simulink model "Project3b"  (R2016a)
settings: Solver=ode5  StartTime=0.0  StopTime=tf  FixedStep=0.001  RelTol=1e-3
values from neighbouring files (symbols this model uses):
  k1 = 1    [Project3_FullCode.m]    (also in Project3a_Code.m = 30; Project3b_Code.m)
  k2 = 1    [Project3_FullCode.m]    (also in Project3a_Code.m = 40; Project3b_Code.m)
  ugain = 1    [Project3_FullCode.m]    (also in Project3a_Code.m; Project3b_Code.m)
  x10 = 0    [Project3_FullCode.m]    (also in Project3a_Code.m = 1; Project3b_Code.m)
  x20 = 2    [Project3_FullCode.m]    (also in Project3a_Code.m = 0; Project3b_Code.m)
settings Model: Creator=Dell  LastModifiedBy=Dell
settings DataIOCC: SaveFormat=Array

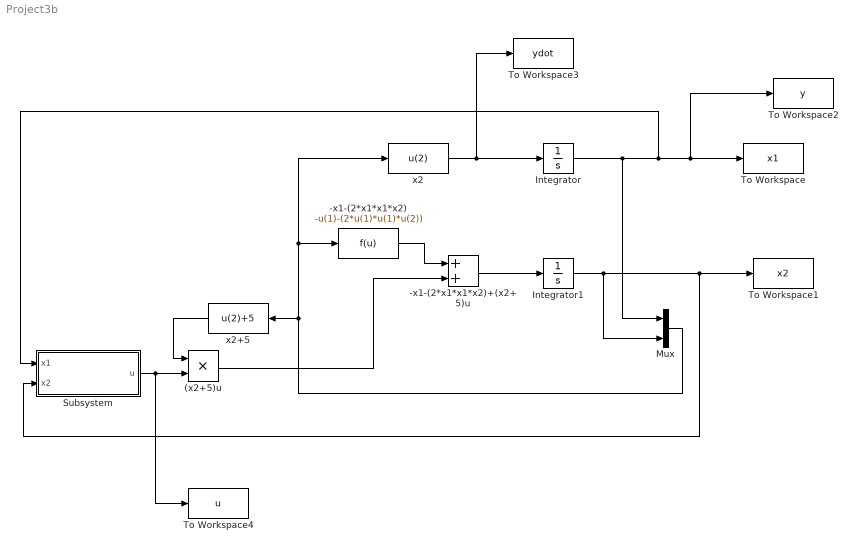
== system Project3b ==
  (x2+5)u : Product
  -x1-(2*x1*x1*x2) : Fcn  Expr=-u(1)-(2*u(1)*u(1)*u(2))
  -x1-(2*x1*x1*x2)+(x2+5)u : Sum
  Integrator : Integrator  InitialCondition=x10
  Integrator1 : Integrator  InitialCondition=x20
  Mux : Mux  Inputs=2
  Subsystem : Subsystem
  To Workspace : ToWorkspace  VariableName=x1  SampleTime=-1
  To Workspace1 : ToWorkspace  VariableName=x2  SampleTime=-1
  To Workspace2 : ToWorkspace  VariableName=y  SampleTime=-1
  To Workspace3 : ToWorkspace  VariableName=ydot  SampleTime=-1
  To Workspace4 : ToWorkspace  VariableName=u  SampleTime=-1
  x2 : Fcn  Expr=u(2)
  x2+5 : Fcn  Expr=u(2)+5
  wires:
  Integrator/1 -> Mux/1, Subsystem/1(x1), To Workspace2/1, To Workspace/1
  Integrator1/1 -> Mux/2, Subsystem/2("x2 "), To Workspace1/1
  Mux/1 -> x2+5/1, -x1-(2*x1*x1*x2)/1, x2/1
  x2/1 -> To Workspace3/1, Integrator/1
  Subsystem/1(u) -> To Workspace4/1, (x2+5)u/2
  x2+5/1 -> (x2+5)u/1
  -x1-(2*x1*x1*x2)/1 -> -x1-(2*x1*x1*x2)+(x2+5)u/1
  (x2+5)u/1 -> -x1-(2*x1*x1*x2)+(x2+5)u/2
  -x1-(2*x1*x1*x2)+(x2+5)u/1 -> Integrator1/1

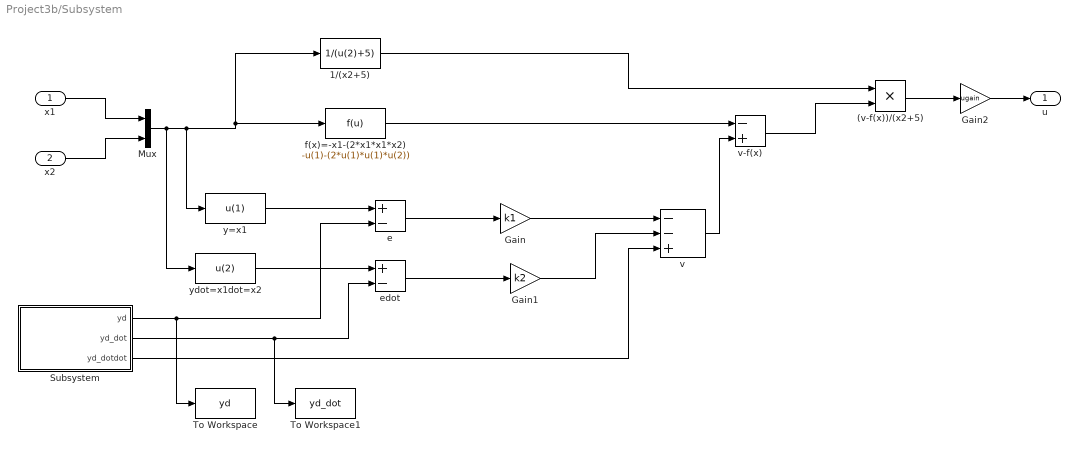
== system Project3b/Subsystem ==
  x1 : Inport
  "x2 " : Inport  Port=2
  (v-f(x))/(x2+5) : Product
  1/(x2+5) : Fcn  Expr=1/(u(2)+5)
  Gain : Gain  Gain=k1
  Gain1 : Gain  Gain=k2
  Gain2 : Gain  Gain=ugain
  Mux : Mux  Inputs=2
  Subsystem : Subsystem
  To Workspace : ToWorkspace  VariableName=yd  SampleTime=-1
  To Workspace1 : ToWorkspace  VariableName=yd_dot  SampleTime=-1
  e : Sum  Inputs=+-
  edot : Sum  Inputs=+-
  f(x)=-x1-(2*x1*x1*x2) : Fcn  Expr=-u(1)-(2*u(1)*u(1)*u(2))
  v : Sum  Inputs=--+
  v-f(x) : Sum  Inputs=-+
  y=x1 : Fcn  Expr=u(1)
  ydot=x1dot=x2 : Fcn  Expr=u(2)
  u : Outport
  wires:
  x1/1 -> Mux/1
  "x2 "/1 -> Mux/2
  Mux/1 -> ydot=x1dot=x2/1, y=x1/1, f(x)=-x1-(2*x1*x1*x2)/1, 1/(x2+5)/1
  y=x1/1 -> e/1
  Subsystem/1(yd) -> e/2, To Workspace/1
  ydot=x1dot=x2/1 -> edot/1
  Subsystem/2(yd_dot) -> To Workspace1/1, edot/2
  e/1 -> Gain/1
  edot/1 -> Gain1/1
  Gain/1 -> v/1
  Gain1/1 -> v/2
  Subsystem/3(yd_dotdot) -> v/3
  f(x)=-x1-(2*x1*x1*x2)/1 -> v-f(x)/1
  v/1 -> v-f(x)/2
  1/(x2+5)/1 -> (v-f(x))/(x2+5)/1
  v-f(x)/1 -> (v-f(x))/(x2+5)/2
  (v-f(x))/(x2+5)/1 -> Gain2/1
  Gain2/1 -> u/1

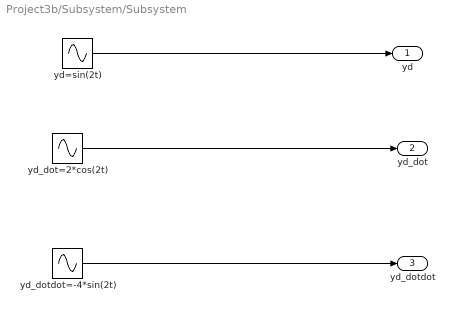
== system Project3b/Subsystem/Subsystem ==
  " yd=sin(2t)" : Sin  Frequency=2  SampleTime=0
  yd_dot=2*cos(2t) : Sin  Amplitude=2  Frequency=2  Phase=pi/2  SampleTime=0
  yd_dotdot=-4*sin(2t) : Sin  Amplitude=-4  Frequency=2  SampleTime=0
  yd : Outport
  yd_dot : Outport  Port=2
  yd_dotdot : Outport  Port=3
  wires:
  " yd=sin(2t)"/1 -> yd/1
  yd_dot=2*cos(2t)/1 -> yd_dot/1
  yd_dotdot=-4*sin(2t)/1 -> yd_dotdot/1
